simulink model "keyboard_2_turtlebot"  (R2020a)
settings: Solver=VariableStepAuto  StartTime=0.0  StopTime=10.0  RelTol=1e-3
settings Model: Creator=grady  LastModifiedBy=grady

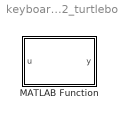
== system keyboard_2_turtlebot ==
  MATLAB Function : MATLAB Function  TreatAsAtomicUnit=on

== matlab function keyboard_2_turtlebot/MATLAB Function ==
  data: u input; y output
function y = ROS_START(u)
rosinit('192.168.1.26')

y = u;
